simulink library "libbha_kinematic"  (R2015b)
settings: Solver=FixedStepDiscrete  StartTime=0.0  StopTime=Inf  FixedStep=0.004  RelTol=1e-3
PostLoadFcn:
  | , if any(exist('dsrtsu_mdlpostloadfcn', 'file') == [2, 3, 6]), try dsrtsu_mdlpostloadfcn('Execute', bdroot); catch fprintf('Error in PostLoadFcn (dsrtsu_mdlpostloadfcn) for model "%s":\n %s\n', bdroot, lasterr); end, end,
undefined symbols (not defined in the file or in its folder): BHA, BHASIM
libraries: libbha_kinematic x14
(part 2 of 3)

== matlab function libbha_kinematic/BHA_Kin_v_vc_SectionX/Section-Kinematics ==
  data: l_Ik input; S_RIh_RIb output; d_Ij input; l_Ib input; l_Ih input; theta_I input size=1; S_RIj_RIb output; T_KImb_Ib input
function [S_RIh_RIb, S_RIj_RIb] = fcn(l_Ik, d_Ij, l_Ib, l_Ih, theta_I, T_KImb_Ib)
%#codegen

ell_Ib  = l_Ib*cos(theta_I);
ell_Ih  = l_Ih*cos(theta_I);

m_I  = size(d_Ij,1)-3;

S_RI0_RIb       = [eye(3),[0;0;ell_Ib]; [0,0,0,1]];
S_RIh_RIm_I     = [eye(3),[0;0;ell_Ih]; [0,0,0,1]];
S_RIj_RIb       = eye(4, 4*(size(d_Ij, 1)));
S_RIj_RIb(:,1:4)= T_KImb_Ib;
S_RIj_RIb(:,5:8)= T_KImb_Ib*S_RI0_RIb;

l_Ijk   = ones(m_I, 1) * (l_Ik./m_I)';
h_Ijk   = abs(sqrt(l_Ijk.^2 - diff(d_Ij(2:end-1, 1)).^2*ones(1,3)));

S_RIh_RIb = S_RI0_RIb;
for jj = 1:m_I
    d_IJ    = d_Ij(jj+2, 1);
    h_IJ1   = h_Ijk(jj, 1);
    h_IJ2   = h_Ijk(jj, 2);
    h_IJ3   = h_Ijk(jj, 3);
    
    ell     = (d_IJ*(h_IJ1+h_IJ2+h_IJ3)) /...
              (2*sqrt(abs(h_IJ1^2+h_IJ2^2+h_IJ3^2 - h_IJ1*h_IJ2-h_IJ1*h_IJ3-h_IJ2*h_IJ3 ))) *...
              asin(2*sqrt(abs(h_IJ1^2+h_IJ2^2+h_IJ3^2 - h_IJ1*h_IJ2-h_IJ1*h_IJ3-h_IJ2*h_IJ3 )) / (3*d_IJ));
    kappa   = (2*sqrt(abs(h_IJ1^2+h_IJ2^2+h_IJ3^2 - h_IJ1*h_IJ2-h_IJ1*h_IJ3-h_IJ2*h_IJ3 ))) / ...
              (d_IJ*(h_IJ1+h_IJ2+h_IJ3));
    phi     = atan2((sqrt(3)*(h_IJ3-h_IJ2)), (h_IJ2+h_IJ3-2*h_IJ1));
    
    if kappa*ell > 1e-6
        S_RIh_RIb = S_RIh_RIb * [(cos(phi))^2*(cos(kappa*ell)-1)+1,     sin(phi)*cos(phi)*(cos(kappa*ell)-1),           cos(phi)*sin(kappa*ell),    cos(phi)*(1-cos(kappa*ell)) / kappa;...
                                 sin(phi)*cos(phi)*(cos(kappa*ell)-1),  (cos(phi))^2*(1-cos(kappa*ell))+cos(kappa*ell), sin(phi)*sin(kappa*ell),    sin(phi)*(1-cos(kappa*ell)) / kappa;...
                                 -cos(phi)*sin(kappa*ell),              -sin(phi)*sin(kappa*ell),                       cos(kappa*ell),             sin(kappa*ell)/kappa;...
                                 0,                                     0,                                              0,                          1                                       ];
    else
        S_RIh_RIb = S_RIh_RIb * [eye(3), [0; 0; mean([h_IJ1,h_IJ2,h_IJ3])]; [0, 0, 0, 1]];
    end
    S_RIj_RIb(:, (1:4)+4*(jj+1)) = T_KImb_Ib*S_RIh_RIb;
end
S_RIh_RIb = S_RIh_RIb*S_RIh_RIm_I;
S_RIj_RIb(:,(1:4)+4*(m_I+2)) = T_KImb_Ib*S_RIh_RIb;

== matlab function libbha_kinematic/BHA_Kin_Dir_CC_cont/DK_ConstCurv ==
  data: h output; q input; H_1b_w input; r_i input; h_ib input; h_ih input; k output
function [h, k]   = f_az2pose(q, H_1b_w, r_i, h_ib, h_ih)
n=3;
% XXXXXXXXXXXXXXXXXXXXXXXXXXXXXXXXXXXXXXXXXXXXXXXXXXXXXXXXXXXXXXXXXXXXXXXXX
% Analytische Berechnung der Transformationen f_allg_kK und f_spez_kK_kA 
% - Modell - Constant Curvature Continuum
%
% Ansatz:
% h     = f_general(k)
% k     = f_specific(q)
%
% mit:
% q     = [ell_11, ell_12, ell_13, ell_21, ell_22, ell_23, ell_31, ell_32, ell_33]
% k     = [phi_1, kappa_1, ell_1, phi_2, kappa_2, ell_2, phi_3, kappa_3, ell_3]
% h     = [ H_1,1,  H_2,1,  H_3,1,  H_1,2,  H_2,2,  H_3,2,  H_1,3,  H_2,3,  H_3,3,  H_1,4,  H_2,4,  H_3,4]
%           1       2       3       4       5       6       7       8       9       10      11      12   
%
% Input:
%   q           [3nx1]  Zustandsvektor der Gelenkkoordinaten (Bogenlänge der Aktoren)
%   H_1b_w      [4x4]   Homogene Transformation: Koordinatensystem 1b
%                       relativ zum Weltsystem
%
% Output:
%   h           [12x1]  Pose des TCP (Homohene Transformation in Vektor geschrieben, ohne Zeile 0,0,0,1)
%   k           [3nx1]  Konfigurationszustand
%
% Parameter:
%   n           [1x1]   Anzahl der Sektionen
%   r_i         [1xn]   Radialer Abstand der Aktoren pro Sektion
%   h_ib        [1xn]   Höhe der Sektionsbasis pro Sektion
%   h_ih        [1xn]   Höhe des Sektionskopfs pro Sektion
%
% Stand: 21.01.2013     Tobias Mahl
% XXXXXXXXXXXXXXXXXXXXXXXXXXXXXXXXXXXXXXXXXXXXXXXXXXXXXXXXXXXXXXXXXXXXXXXXX

    % Direkte Kinematik
    k = f_spez_kK_kA(n, q, r_i);
    [H_nh_w, H_ih_ib] = f_allg_kK(n, k, h_ib, h_ih, H_1b_w);
    h = H2h(H_nh_w);
    
end

%% Allgemeines

function h = H2h(H)
% Transformation:
%   homogene Transformation H --> vektorielle Repräsentation h
%                     H {4x4} --> h {12x1}

    h = reshape(H(1:3,:), [12,1]);
end

function H = h2H(h)
% Transformation:
%   vektorielle Repräsentation h --> homogene Transformation H
%                       h {12x1} --> H {4x4}

    H = [reshape(h, [3,4]); 0,0,0,1];
end

%% XXXXXXXXXXXXXXXXXXXXXXXXXXXXXX f_spez XXXXXXXXXXXXXXXXXXXXXXXXXXXXXXXXXX
function k = f_spez_kK_kA(n, q, r_i)
% Berechnung der Transformation
% Aktorbogenlängen q --> Konfigurationszustand k  
% des kontinuierlichen Roboters gemäß der Abbildung:
% k = f_specific(q)
% 
% Input:
%   q  [3nx1]   Aktorbogenlängen (kontinuierlich biegender Aktor)
%
% Output:
%   k     [3nx1]   Konfigurationszustand mit (phi_i, kappa_i, ell_i)
%
% Parameter:
%   r_i     [1xn]   Radiale Abständ der Aktoren je Sektion i
    
    k = zeros(3*n, 1);
    for ii=1:n
        k((1:3)+(ii-1)*3, 1) = f_spez_kK_kA_I(q((1:3)+(ii-1)*3, 1), r_i(ii));
    end
end

function k_I = f_spez_kK_kA_I(q_I, r_I)
% Berechnung der Transformation
% Aktorbogenlängen q_I --> Konfigurationszustand [phi_I, kappa_I, ell_I]  
% einer einzelnen Sektion gemäß der Abbildung:
% k_I = f_specific_I(q_I)
% 
% Input:
%   q_I  [3x1]   Aktorbogenlängen (kontinuierlich biegender Aktor)
%
% Output:
%   k_I     [3x1]   Konfigurationszustand (phi_I, kappa_I, ell_I)
%
% Parameter:
%   r_I     [1x1]   Radialer Abstand der Aktoren

    wurzel = sqrt(max([0, q_I(1,1)^2 + q_I(2,1)^2 + q_I(3,1)^2 - q_I(1,1)*q_I(2,1) - q_I(1,1)*q_I(3,1) - q_I(2,1)*q_I(3,1)]));
    
    phi_I  = atan2(sqrt(3)*(q_I(3,1)-q_I(2,1)), q_I(2,1)+q_I(3,1)-2*q_I(1,1));
    kappa_I= 2*wurzel / (r_I*(q_I(1,1)+q_I(2,1)+q_I(3,1)));
    ell_I  = (q_I(1,1)+q_I(2,1)+q_I(3,1))/3;
    
    k_I    = [phi_I; kappa_I; ell_I];
end

%% XXXXXXXXXXXXXXXXXXXXXXXXXXXXXX f_allg XXXXXXXXXXXXXXXXXXXXXXXXXXXXXXXXXX
function [H_nh_w, H_ih_ib] = f_allg_kK(n, k, h_ib, h_ih, H_1b_w)

% Berechnung der homogenen Transformation der I-ten Sektion gemäß Abbildung
% H = f_general_H(k, h_ib, h_ih, H_1b_w)
% 
% Input:
%   k       Konfigurationszustand (phi_i, kappa_i, ell_i) aller Sektionen
%   h_ib    Höhen der Sektionsfüsse (Sektionen i)
%   h_ih    Höhen des Sektionsköpfe (Sektionen i)
%
% Output:   
%   H_nh_w  Homogene Transformation zwischen n-tem Kopf- und Welt-Koordinatensystem

    H_nh_w  = H_1b_w;
    H_ih_ib = zeros(4, 4, n);
    
    for ii = 1:n
        H_Ih_Ib         = f_allg_kK_I(k((1:3)+(ii-1)*3, 1), h_ib(ii), h_ih(ii));
        H_nh_w          = H_nh_w*H_Ih_Ib;
        H_ih_ib(:,:,ii) = H_Ih_Ib;
    end
end

function H_Ih_Ib = f_allg_kK_I(k_I, h_Ib, h_Ih)

% Berechnung der homogenen Transformation der I-ten Sektion gemäß Abbildung
% H_I = f_general_H_I(k_I, h_Ib, h_Ih)
% 
% Input:
%   k       Konfigurationszustand (phi_I, kappa_I, ell_I) der Sektion I
%   h_Ib    Höhe der Sektionsbasis (Sektion I)
%   h_Ih    Höhe des Sektionskopfs (Sektion I)
%
% Output:   
%   H_Ih_Ib Homogene Transformation zwischen Kopf- und Basis-Koordinatensystem

    %% homogene Transformation der Basis
    H_I0_Ib = [eye(3), [0; 0; h_Ib];...
               0,0,0,  1];

    %% homogene Transformation des Kopfs
    H_Ih_I1 = [eye(3), [0; 0; h_Ih];...
               0,0,0,  1];

    %% homogene Transformation des Aktorbereichs
    eps =   1e-7;
    
    % Berechnung gemäß lim kappa->0 (Biegelinie ist eine Gerade)
    if(k_I(2) < eps)
        R_I1_I0 = eye(3);
        o_I1_I0 = [0; 0; k_I(3)];

    % Berechnung gemäß kappa>0 (Biegelinie ist ein Kreissegment)
    else
        s_phi   = sin(k_I(1));
        c_phi   = cos(k_I(1));
        s_kl    = sin(k_I(2)*k_I(3));
        c_kl    = cos(k_I(2)*k_I(3));

        R_I1_I0 = [c_phi^2*(c_kl-1)+1,      s_phi*c_phi*(c_kl-1),       c_phi*s_kl;...
                   s_phi*c_phi*(c_kl-1),    c_phi^2*(1-c_kl)+c_kl,      s_phi*s_kl;...
                   -c_phi*s_kl,             -s_phi*s_kl,                c_kl];

        o_I1_I0 = [c_phi*(1-c_kl)/k_I(2);...
                   s_phi*(1-c_kl)/k_I(2);...
                   s_kl/k_I(2)];
    end
    H_I1_I0 = [R_I1_I0, o_I1_I0;...
               0,0,0,   1];

    H_Ih_Ib = H_I0_Ib*H_I1_I0*H_Ih_I1;
end

== matlab function libbha_kinematic/J_task_5DoF/J_task_5DoF ==
  data: h input; J output size=[5,12]
function J    = J_task_5DoF(h)
% XXXXXXXXXXXXXXXXXXXXXXXXXXXXXXXXXXXXXXXXXXXXXXXXXXXXXXXXXXXXXXXXXXXXXXXXX
% Analytische Berechnung der taskspezifischen Jacobi-Matrix
%
% Ansatz:
% x         = f_task(h)
% J_task    = dx / dh
%
% mit:
% x         = [x, y, z, tx, ty]^T = [h_10, h_11, h12, atan(h8/h9), -atan(h7/h9)]^T
% h         = [ H_1,1,  H_2,1,  H_3,1,  H_1,2,  H_2,2,  H_3,2,  H_1,3,  H_2,3,  H_3,3,  H_1,4,  H_2,4,  H_3,4]
%               1       2       3       4       5       6       7       8       9       10      11      12   
%
% Task variables:
%   x                   x-Position
%   y                   y-Position
%   z                   z-Position
%   theta_x             Winkel um x-Achse(w) der Projektion des Vektors ([0;0;1] in nh)
%   theta_y             Winkel um y-Achse(w) der Projektion des Vektors ([0;0;1] in nh)
%
% Input:
%   h           [12x1]  Pose des TCP relativ zum Task-Koordinatensystem
%
% Output:
%   J_task_xyz  [5x12]  Task-spezifische Jacobi-Matrix
%
% Parameter:
%
% Stand: 21.01.2013     Tobias Mahl
% XXXXXXXXXXXXXXXXXXXXXXXXXXXXXXXXXXXXXXXXXXXXXXXXXXXXXXXXXXXXXXXXXXXXXXXXX

J      = zeros(5, 12);

J(1,10)= 1;
J(2,11)= 1;
J(3,12)= 1;

J(4,8) = -h(9)/(h(9)^2+h(8)^2);
J(4,9) =  h(8)/(h(9)^2+h(8)^2);

J(5,7) =  h(9)/(h(9)^2+h(7)^2);
J(5,9) = -h(7)/(h(9)^2+h(7)^2);

== matlab function libbha_kinematic/f_task5DoF/f_task5DoF ==
  data: h input; x output
function x = f_task_5Dof(h)

x = [h(10);
     h(11);
     h(12);
     -atan2(h(8), h(9));
     atan2(h(7), h(9))];

== matlab function libbha_kinematic/BHA_Kin_DirDiff_1stO_CC_cont/J_general & J_specific ==
  data: h output; k output; q input; H_1b_w input; J_allg_kK output; r_i input; h_ib input; h_ih input; J_spez_kK_kA output
function [h, k, J_allg_kK, J_spez_kK_kA] = Jacobi_CC_continuum(q, H_1b_w, r_i, h_ib, h_ih)
n = 3; % Parameter
% XXXXXXXXXXXXXXXXXXXXXXXXXXXXXXXXXXXXXXXXXXXXXXXXXXXXXXXXXXXXXXXXXXXXXXXXX
% Analytische Berechnung der Jacobi-Matrizen J_general und J_specific 
% - Modell - Constant Curvature Continuum
%
% Ansatz:
% h     = f_general(k)
% k     = f_specific(q)
% ==>
% h     = f_general(f_specific(q))
%
% J_general     = dh / dk
% J_specific    = dk / dq
%
% mit:
% q     = [ell_11, ell_12, ell_13, ell_21, ell_22, ell_23, ell_31, ell_32, ell_33]
% k     = [phi_1, kappa_1, ell_1, phi_2, kappa_2, ell_2, phi_3, kappa_3, ell_3]
% h     = [ H_1,1,  H_2,1,  H_3,1,  H_1,2,  H_2,2,  H_3,2,  H_1,3,  H_2,3,  H_3,3,  H_1,4,  H_2,4,  H_3,4]
%           1       2       3       4       5       6       7       8       9       10      11      12   
%
% Input:
%   q           [3nx1]  Zustandsvektor der Gelenkkoordinaten (Bogenlänge der Aktoren)
%   H_1b_w   [4x4]   Homogene Transformation: Koordinatensystem 1b
%                       relativ zum Weltsystem
%
% Output:
%   h           [12x1]  Pose des TCP (Homohene Transformation in Vektor geschrieben, ohne Zeile 0,0,0,1)
%   J_general   [12x3n] Allgemeingültige Jacobi-Matrix für kontinuierliche Manipulatoren
%   k           [3nx1]  Konfigurationszustand
%   J_specific  [3nx3n] Manipulator-spezifische Jacobimatrix (3-Aktuator Kontinuum Manipulator)
%
% Parameter:
%   n           [1x1]   Anzahl der Sektionen
%   r_i         [1xn]   Radialer Abstand der Aktoren pro Sektion
%   h_ib        [1xn]   Höhe der Sektionsbasis pro Sektion
%   h_ih        [1xn]   Höhe des Sektionskopfs pro Sektion
%
% Stand: 21.01.2013     Tobias Mahl
% XXXXXXXXXXXXXXXXXXXXXXXXXXXXXXXXXXXXXXXXXXXXXXXXXXXXXXXXXXXXXXXXXXXXXXXXX
    
    % Direkte Kinematik
    eps_kappa_i_dK = 1e-7*ones(1, n);
    
    k = f_spez_kK_kA(n, q, r_i);
    %[H_nh_w, H_ih_ib] = f_allg_kK(n, k, h_ib, h_ih, H_1b_w, eps_kappa_i_dK);
    [H_nh_w, ~] = f_allg_kK(n, k, h_ib, h_ih, H_1b_w, eps_kappa_i_dK);
    h = H2h(H_nh_w);
    
    % Direkte Differentielle Kinematik
    eps_kappa_i_ddK = 5e-4*ones(1, n);
    eps_kappa_i_ddK = max(eps_kappa_i_ddK, 1.01*eps_kappa_i_dK); %eps_kappa_i_ddK !> eps_kappa_i_dK
        
    % Regularisierung
    [q_reg, k_reg] = regularisierung(n, q, k, r_i, eps_kappa_i_ddK);
    %[H_nh_w_reg, H_ih_ib_reg] = f_allg_kK(n, k_reg, h_ib, h_ih, H_1b_w, eps_kappa_i_dK);
    [~, H_ih_ib_reg] = f_allg_kK(n, k_reg, h_ib, h_ih, H_1b_w, eps_kappa_i_dK);
    
    % Direkte differentielle Kinematik 1. Ordnung
    J_spez_kK_kA = df_spez_kK_kA_dq(n, q_reg, r_i);
    %[J_allg_kK, dh_Ih_Ib_dk_I_all] = df_allg_kK_dk(n, k_reg, h_ib, h_ih, H_1b_w, H_ih_ib_reg, eps_kappa_i_ddK.*0.8);
    [J_allg_kK, ~] = df_allg_kK_dk(n, k_reg, h_ib, h_ih, H_1b_w, H_ih_ib_reg, eps_kappa_i_ddK.*0.8);
end


%% XXXXXXXXXXXXXXXXXXXXXX Regularisierung XXXXXXXXXXXXXXXXXXXXXXXXXXXXXXXXX
function [q_reg, k_reg] = regularisierung(n, q, k, r_i, eps_kappa)

    q_reg = q;
    k_reg = k;
    
    for ii = 1:n
        k_I         = k((1:3)+3*(ii-1));
        r_I         = r_i(ii);
        eps_kappa_I = eps_kappa(ii);
        
        if (k_I(2) < eps_kappa_I)
            q_reg((1:3)+3*(ii-1)) = k_I(3) - eps_kappa_I*k_I(3)*r_I*cos(2*pi/3*[0;1;2]-k_I(1));
            k_reg((1:3)+3*(ii-1)) = f_spez_kK_kA_I(q_reg((1:3)+3*(ii-1)), r_I);
        end
    end
end

%% XXXXXXXXXXXXXXXXXXXXXXXXXXXXXX Allgemeines XXXXXXXXXXXXXXXXXXXXXXXXXXXXX
function h = H2h(H)
% Transformation:
%   homogene Transformation H --> vektorielle Repräsentation h
%                     H {4x4} --> h {12x1}

    h = reshape(H(1:3,:), [12,1]);
end

function H = h2H(h)
% Transformation:
%   vektorielle Repräsentation h --> homogene Transformation H
%                       h {12x1} --> H {4x4}

    H = [reshape(h, [3,4]); 0,0,0,1];
end

function [H_2_in_0] = clc_Trafo_H(H_1_in_0, H_2_in_1)
% Input:
%   - Eine Matrix [4x4]
%   - Eine Matrix [4*nz x 4*ns]
%
% Output:
%   - H_2_in_0 [4*nz x 4*ns] = H_1_in_0*H_2_in_1

    [nz1, ns1] = size(H_1_in_0);
    [nz2, ns2] = size(H_2_in_1);

    nz_max = max(nz1./4, nz2./4);
    ns_max = max(ns1./4, ns2./4);

    H_2_in_0 = zeros(4*nz_max, 4*ns_max);

    if (nz1+ns1) < (nz2+ns2)
        for zz = 1:nz_max
            for ss = 1:ns_max
                H_2_in_0((1:4)+4*(zz-1), (1:4)+4*(ss-1)) = H_1_in_0 * H_2_in_1((1:4)+4*(zz-1), (1:4)+4*(ss-1));
            end
        end
    else
        for zz = 1:nz_max
            for ss = 1:ns_max
                H_2_in_0((1:4)+4*(zz-1), (1:4)+4*(ss-1)) = H_1_in_0((1:4)+4*(zz-1), (1:4)+4*(ss-1)) * H_2_in_1;
            end
        end
    end
end

%% XXXXXXXXXXXXXXXXXXXXXXXXXXXXXX f_spez XXXXXXXXXXXXXXXXXXXXXXXXXXXXXXXXXX
function k = f_spez_kK_kA(n, q, r_i)
% Berechnung der Transformation
% Aktorbogenlängen q --> Konfigurationszustand k  
% des kontinuierlichen Roboters gemäß der Abbildung:
% k = f_specific(q)
% 
% Input:
%   q  [3nx1]   Aktorbogenlängen (kontinuierlich biegender Aktor)
%
% Output:
%   k     [3nx1]   Konfigurationszustand mit (phi_i, kappa_i, ell_i)
%
% Parameter:
%   r_i     [1xn]   Radiale Abständ der Aktoren je Sektion i
    
    k = zeros(3*n, 1);
    for ii=1:n
        k((1:3)+(ii-1)*3, 1) = f_spez_kK_kA_I(q((1:3)+(ii-1)*3, 1), r_i(ii));
    end
end

function k_I = f_spez_kK_kA_I(q_I, r_I)
% Berechnung der Transformation
% Aktorbogenlängen q_I --> Konfigurationszustand [phi_I, kappa_I, ell_I]  
% einer einzelnen Sektion gemäß der Abbildung:
% k_I = f_specific_I(q_I)
% 
% Input:
%   q_I  [3x1]   Aktorbogenlängen (kontinuierlich biegender Aktor)
%
% Output:
%   k_I     [3x1]   Konfigurationszustand (phi_I, kappa_I, ell_I)
%
% Parameter:
%   r_I     [1x1]   Radialer Abstand der Aktoren

    q_dist = max([0, q_I(1,1)^2 + q_I(2,1)^2 + q_I(3,1)^2 - q_I(1,1)*q_I(2,1) - q_I(1,1)*q_I(3,1) - q_I(2,1)*q_I(3,1)]);
    
    phi_I  = atan2(sqrt(3)*(q_I(3,1)-q_I(2,1)), q_I(2,1)+q_I(3,1)-2*q_I(1,1));
    kappa_I= 2*sqrt(q_dist) / (r_I*(q_I(1,1)+q_I(2,1)+q_I(3,1)));
    ell_I  = (q_I(1,1)+q_I(2,1)+q_I(3,1))/3;
    
    k_I    = [phi_I; kappa_I; ell_I];
end

%% XXXXXXXXXXXXXXXXXXXXXXXXXXXXXX f_allg XXXXXXXXXXXXXXXXXXXXXXXXXXXXXXXXXX
function [H_nh_w, H_ih_ib] = f_allg_kK(n, k, h_ib, h_ih, H_1b_w, eps_kappa_i)
% Berechnung der homogenen Transformation der I-ten Sektion gemäß Abbildung
% H = f_general_H(k, h_ib, h_ih, H_1b_w)
% 
% Input:
%   k           Konfigurationszustand (phi_i, kappa_i, ell_i) aller Sektionen
%   h_ib        Höhen der Sektionsfüsse (Sektionen i)
%   h_ih        Höhen des Sektionsköpfe (Sektionen i)
%   eps_kappa_i Minimale Krümmung für die ungleich Gerade gerechnet wird (Sektionen i)
%
% Output:   
%   H_nh_w  Homogene Transformation zwischen n-tem Kopf- und Welt-Koordinatensystem

    H_nh_w  = H_1b_w;
    H_ih_ib = zeros(4, 4, n);
    
    for ii = 1:n
        H_Ih_Ib         = f_allg_kK_I(k((1:3)+(ii-1)*3, 1), h_ib(ii), h_ih(ii), eps_kappa_i(ii));
        H_nh_w          = H_nh_w*H_Ih_Ib;
        H_ih_ib(:,:,ii) = H_Ih_Ib;
    end
end

function H_Ih_Ib = f_allg_kK_I(k_I, h_Ib, h_Ih, eps_kappa_I)
% Berechnung der homogenen Transformation der I-ten Sektion gemäß Abbildung
% H_I = f_general_H_I(k_I, h_Ib, h_Ih)
% 
% Input:
%   k           Konfigurationszustand (phi_I, kappa_I, ell_I) der Sektion I
%   h_Ib        Höhe der Sektionsbasis (Sektion I)
%   h_Ih        Höhe des Sektionskopfs (Sektion I)
%   eps_kappa_I Minimale Krümmung für die ungleich Gerade gerechnet wird (Sektione I)
%
% Output:   
%   H_Ih_Ib Homogene Transformation zwischen Kopf- und Basis-Koordinatensystem

    % homogene Transformation der Basis
    H_I0_Ib = [eye(3), [0; 0; h_Ib];...
               0,0,0,  1];

    % homogene Transformation des Kopfs
    H_Ih_I1 = [eye(3), [0; 0; h_Ih];...
               0,0,0,  1];

    % homogene Transformation des Aktorbereichs
    % Berechnung gemäß lim kappa->0 (Biegelinie ist eine Gerade)
    if(k_I(2) < eps_kappa_I)
        R_I1_I0 = eye(3);
        o_I1_I0 = [0; 0; k_I(3)];

    % Berechnung gemäß kappa>0 (Biegelinie ist ein Kreissegment)
    else
        s_phi   = sin(k_I(1));
        c_phi   = cos(k_I(1));
        s_kl    = sin(k_I(2)*k_I(3));
        c_kl    = cos(k_I(2)*k_I(3));

        R_I1_I0 = [c_phi^2*(c_kl-1)+1,      s_phi*c_phi*(c_kl-1),       c_phi*s_kl;...
                   s_phi*c_phi*(c_kl-1),    c_phi^2*(1-c_kl)+c_kl,      s_phi*s_kl;...
                   -c_phi*s_kl,             -s_phi*s_kl,                c_kl];

        o_I1_I0 = [c_phi*(1-c_kl)/k_I(2);...
                   s_phi*(1-c_kl)/k_I(2);...
                   s_kl/k_I(2)];
    end
    H_I1_I0 = [R_I1_I0, o_I1_I0;...
               0,0,0,   1];

    H_Ih_Ib = H_I0_Ib*H_I1_I0*H_Ih_I1;
end

%% XXXXXXXXXXXXXXXXXXXXXXX J_spez XXXXXXXXXXXXXXXXXXXXXXXXXXXXXXXXXXXXXXXXX
function [J_spez_kK_kA] = df_spez_kK_kA_dq(n, q, r_i)
% Jakobimatrix der Trafo: Actuator space --> Configuration Space
% dk/dq  = J_specific(q)
% mit:
% k     = [phi_1, kappa_1, ell_1, phi_2, kappa_2, ell_2, phi_3, kappa_3, ell_3]
% q     = [ell_11, ell_12, ell_13, ell_21, ell_22, ell_23, ell_31, ell_32, ell_33]

    J_spez_kK_kA    = zeros(3*n, 3*n);
    for ii = 1:n
        q_I = q((1:3)+3*(ii-1), 1);
        r_I = r_i(ii);

        J_spez_kK_kA((1:3)+3*(ii-1), (1:3)+3*(ii-1)) = df_spez_kK_kA_dq_I(q_I, r_I);
    end
end

function J_spez_kK_kA_I = df_spez_kK_kA_dq_I(q_I, r_I)
% Berechnung der Jacobimatrix der Transformation
% Aktorbogenlängen q_I --> Konfigurationszustand [phi_I, kappa_I, ell_I]  
% einer einzelnen Sektion gemäß der Abbildung:
% dk_I / dq_I = df_spez_kK_kA_dq_I(q_I)
% 
% Input:
%   q_I  [3x1]   Aktorbogenlängen (kontinuierlich biegender Aktor)
%
% Output:
%   df_spez_kK_kA_dq_I    [3x3]   Jacobimatrix einer Sektion
%
% Parameter:
%   r_I     [1x1]   Radialer Abstand der Aktoren

    % Vermeidung Singularität (Wenn Output geschrieben wird, dann Ergebnis nicht korrekt!)
    eps_q_dist  = eps;
    eps_q1      = 1e-5;
    q_dist      = max(0, q_I(1,1)^2 + q_I(2,1)^2 + q_I(3,1)^2 - q_I(1,1)*q_I(2,1) - q_I(1,1)*q_I(3,1) - q_I(2,1)*q_I(3,1));
    while (q_dist<eps_q_dist)
        q_I(1,1)= q_I(1,1)-eps_q1;
        q_dist  = max(0, q_I(1,1)^2 + q_I(2,1)^2 + q_I(3,1)^2 - q_I(1,1)*q_I(2,1) - q_I(1,1)*q_I(3,1) - q_I(2,1)*q_I(3,1));
        %q_dist_ddk1 = q_dist;
    end
    
    % Substitution
    q_sum  = (q_I(1,1)+q_I(2,1)+q_I(3,1));

    % Partielle Ableitungen
    d_phi_dell1     =  sqrt(3)/2*(q_I(3,1)-q_I(2,1)) / q_dist;
    d_phi_dell2     = -sqrt(3)/2*(q_I(3,1)-q_I(1,1)) / q_dist;
    d_phi_dell3     =  sqrt(3)/2*(q_I(2,1)-q_I(1,1)) / q_dist;
    
    d_kappa_dell1   = 3*(q_I(1,1)*q_I(2,1) + q_I(1,1)*q_I(3,1) - q_I(2,1)^2 - q_I(3,1)^2) / (sqrt(q_dist)*r_I*q_sum^2);
    d_kappa_dell2   = 3*(q_I(1,1)*q_I(2,1) + q_I(2,1)*q_I(3,1) - q_I(1,1)^2 - q_I(3,1)^2) / (sqrt(q_dist)*r_I*q_sum^2);
    d_kappa_dell3   = 3*(q_I(1,1)*q_I(3,1) + q_I(2,1)*q_I(3,1) - q_I(1,1)^2 - q_I(2,1)^2) / (sqrt(q_dist)*r_I*q_sum^2);

    d_ell_dell1     = 1/3;
    d_ell_dell2     = 1/3;
    d_ell_dell3     = 1/3;
    
    
    J_spez_kK_kA_I  = [d_phi_dell1,    d_phi_dell2,    d_phi_dell3;
                       d_kappa_dell1,  d_kappa_dell2,  d_kappa_dell3
                       d_ell_dell1,    d_ell_dell2,    d_ell_dell3   ];
end

%% XXXXXXXXXXXXXXXXXXXXXXX J_allg XXXXXXXXXXXXXXXXXXXXXXXXXXXXXXXXXXXXXXXXX
function [J_allg_kK, dh_Ih_Ib_dk_I_all]  = df_allg_kK_dk(n, k, h_ib, h_ih, H_1b_w, H_ih_ib, eps_kappa_i)
% Funktion zur Berechnung der Jacobimatrix eines Continuum Manipulators
%
% Trafo: Configuration Space --> Task Space
% h = f_general(k)
%
% h     = [ H_1,1,  H_2,1,  H_3,1,  H_1,2,  H_2,2,  H_3,2,  H_1,3,  H_2,3,  H_3,3,  H_1,4,  H_2,4,  H_3,4]
%           1       2       3       4       5       6       7       8       9       10      11      12   
% k     = [phi_1, kappa_1, ell_1, phi_2, kappa_2, ell_2, phi_3, kappa_3, ell_3]
%

    J_allg_kK           = zeros(12, 3*n);
    dh_Ih_Ib_dk_I_all   = zeros(12, 3*n); % = [df_allg_kK_1_dk_11 ... df_allg_kK_n_dk_n3]
    for ii = 1:n
        % Ableitungstensor der I-ten Sektion
        dH_Ih_Ib_dk_I = df_allg_kK_dk_I(k((1:3)+3*(ii-1), 1), h_ib(ii), h_ih(ii), eps_kappa_i(ii));
        dh_Ih_Ib_dk_I_all(:, (1:3)+3*(ii-1)) = [H2h(dH_Ih_Ib_dk_I(:,:,1)),...
                                                H2h(dH_Ih_Ib_dk_I(:,:,2)),...
                                                H2h(dH_Ih_Ib_dk_I(:,:,3))];
        
        % Ableitungstensor des TCP nach den Konfigurationsparametern der I-ten Sektion 
        dH_nh_w_dk_I = zeros(4,4,3);
        
        % Ableitungsregel dH/dk_IJ = H_1b_w * H_I-1h_in_1b * dH_Ih_in_Ib/dk_IJ * H_nh_in_I+1b 
        H_Imh_1b = eye(4);
        for xi = 1:ii-1
            H_Imh_1b = H_Imh_1b*H_ih_ib(:,:,xi);
        end
        H_nh_Ipb = eye(4);
        for xi = ii+1:n
            H_nh_Ipb = H_nh_Ipb*H_ih_ib(:,:,xi);
        end
        
        dH_nh_w_dk_I(:,:,1) = H_1b_w*H_Imh_1b* dH_Ih_Ib_dk_I(:,:,1) *H_nh_Ipb;
        dH_nh_w_dk_I(:,:,2) = H_1b_w*H_Imh_1b* dH_Ih_Ib_dk_I(:,:,2) *H_nh_Ipb;
        dH_nh_w_dk_I(:,:,3) = H_1b_w*H_Imh_1b* dH_Ih_Ib_dk_I(:,:,3) *H_nh_Ipb;
        
        % Jacobimatrix
        J_allg_kK(:, (1:3)+3*(ii-1)) = [H2h(dH_nh_w_dk_I(:,:,1)),...
                                        H2h(dH_nh_w_dk_I(:,:,2)),...
                                        H2h(dH_nh_w_dk_I(:,:,3))];
    end
end

function dH_Ih_Ib_dk_I = df_allg_kK_dk_I(k_I, h_Ib, h_Ih, eps_kappa_I)
% Berechnung des Ableitungstensors der homogenen Transformation der I-ten Sektion S_Ih_in_Ib
% 
% Input:
%   k           Konfigurationszustand (phi_I, kappa_I, ell_I) der Sektion I
%   h_Ib        Höhe der Sektionsbasis (Sektion I)
%   h_Ih        Höhe des Sektionskopfs (Sektion I)
%
% Output:   
%   dH_Ih_Ib_dk_I   Ableitungstensor [4x4x3] der homogenen Transformation zwischen Kopf- und Fuß-Koordinatensystem

    %% homogene Transformation des Fußes
    H_I0_Ib = [eye(3), [0; 0; h_Ib];...
               0,0,0,  1];

    %% homogene Transformation des Kopfs
    H_Ih_I1 = [eye(3), [0; 0; h_Ih];...
               0,0,0,  1];
           
    %% homogene Transformation des Aktorbereichs
    % Ableitungstensor
    dH_Ih_Ib_dk_I = zeros(4,4,3);
    
    % Regularisierung (Wenn Output geschrieben wird, dann Ergebnis nicht korrekt!)
    if k_I(2) < eps_kappa_I
        k_I(2) = eps_kappa_I;
        %kappa_I_ddk1 = k_I(2);
    end

    % Berechnung gemäß kappa>0 (Biegelinie ist ein Kreissegment)
    s_phi   = sin(k_I(1));
    c_phi   = cos(k_I(1));
    s_kl    = sin(k_I(2)*k_I(3));
    c_kl    = cos(k_I(2)*k_I(3));

    % Ableitung der Homogenen Trafo nach dphi_I
    d_H_I1_I0_dphi   = [-2*s_phi*c_phi*(c_kl-1),            c_phi^2*(c_kl-1)-s_phi^2*(c_kl-1),  -s_phi*s_kl,    -s_phi*(1-c_kl)/k_I(2);
                        c_phi^2*(c_kl-1)-s_phi^2*(c_kl-1),  -2*c_phi*(1-c_kl)*s_phi,            c_phi*s_kl,     c_phi*(1-c_kl)/k_I(2);
                        s_phi*s_kl,                         -c_phi*s_kl,                        0,              0;
                        0,                                  0,                                  0,              0                           ];

    dH_Ih_Ib_dk_I(:,:,1) = H_I0_Ib * d_H_I1_I0_dphi * H_Ih_I1;

    % Ableitung der Homogenen Trafo nach dkappa_I
    d_H_I1_I0_dkappa = [-c_phi^2*s_kl*k_I(3),            -s_phi*c_phi*s_kl*k_I(3),                c_phi*c_kl*k_I(3),   c_phi*s_kl*k_I(3)/k_I(2) - c_phi*(1-c_kl)/k_I(2)^2;
                        -s_phi*c_phi*s_kl*k_I(3),        c_phi^2*s_kl*k_I(3) - s_kl*k_I(3),       s_phi*c_kl*k_I(3),   s_phi*s_kl*k_I(3)/k_I(2) - s_phi*(1-c_kl)/k_I(2)^2;
                        -c_phi*c_kl*k_I(3),              -s_phi*c_kl*k_I(3),                      -s_kl*k_I(3),        c_kl*k_I(3)/k_I(2) - s_kl/k_I(2)^2;
                        0,                               0,                                       0,                   0                                                   ];

    dH_Ih_Ib_dk_I(:,:,2) = H_I0_Ib * d_H_I1_I0_dkappa * H_Ih_I1;

    % Ableitung der Homogenen Trafo nach dell_I
    d_H_I1_I0_dell   = [-c_phi^2*s_kl*k_I(2),          -s_phi*c_phi*s_kl*k_I(2),              c_phi*c_kl*k_I(2), c_phi*s_kl;
                        -s_phi*c_phi*s_kl*k_I(2),      c_phi^2*s_kl*k_I(2) - s_kl*k_I(2),     s_phi*c_kl*k_I(2), s_phi*s_kl;
                        -c_phi*c_kl*k_I(2),            -s_phi*c_kl*k_I(2),                    -s_kl*k_I(2),      c_kl;
                        0,                              0,                                      0,                  0           ];

    dH_Ih_Ib_dk_I(:,:,3) = H_I0_Ib * d_H_I1_I0_dell * H_Ih_I1;
end
